simulink model "task4_final"  (R2019b)
settings: Solver=ode45  StartTime=0.0  StopTime=10.0  RelTol=1e-3  EnableMultiTasking=on
settings Model: Creator=Knut  LastModifiedBy=FFARHANW
settings DataIOCC: LimitDataPoints=on  SaveFormat=Array  SignalLoggingSaveFormat=ModelDataLogs  ReturnWorkspaceOutputs=off
settings OptimizationCC: BlockReduction=off  BooleanDataType=off
settings DebuggingCC: SaveWithParameterizedLinksMsg=none  UnderspecifiedInitializationDetection=Classic  MergeDetectMultiDrivingBlocksExec=none  SignalResolutionControl=TryResolveAllWithWarning  MultiTaskDSMMsg=warning  MultiTaskCondExecSysMsg=none  ArithmeticOperatorsInVariantConditions=warning
settings HardwareCC: TargetUnknown=on
settings ModelReferenceCC: PropagateSignalLabelsOutOfModel=off
settings SFSimCC: SimUseLocalCustomCode=off  CustomCodeUndefinedFunction=UseInterfaceOnly
settings RTWCC: RTWUseLocalCustomCode=off
settings CodeAppCC: StateflowObjectComments=on
settings GRTTargetCC: TargetLangStandard=C89/C90 (ANSI)  CombineOutputUpdateFcns=off  GRTInterface=on
settings ConfigComp: CovHtmlReporting=on  CovSaveCumulativeToWorkspaceVar=on  CovSaveSingleToWorkspaceVar=on  CovExternalEMLEnable=off

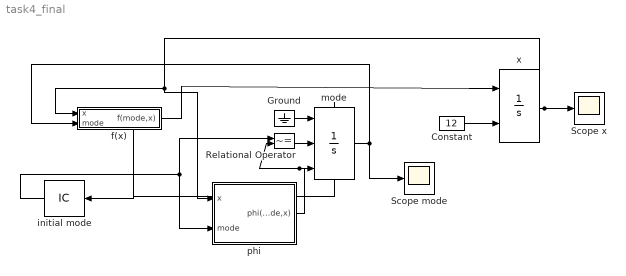
== system task4_final ==
  Constant : Constant  Value=12
  Ground : Ground
  Relational Operator : RelationalOperator  Operator=~=  RndMeth=Nearest  InputSameDT=on
  Scope mode : Scope
  Scope x : Scope
  f(x) : Subsystem  Description=f(x)
  initial mode : InitialCondition
  mode : Integrator  ExternalReset=rising  InitialConditionSource=external  ShowStatePort=on  ZeroCross=off
  phi : Subsystem  Description=f(x)
  x : Integrator  InitialConditionSource=external  LowerSaturationLimit=0
  wires:
  f(x)/1(f(mode,x)) -> x/1
  Ground/1 -> mode/1
  mode/State -> initial mode/1
  initial mode/1 -> phi/2(mode), Relational Operator/1
  mode/1 -> Scope mode/1, f(x)/2(mode)
  phi/1(phi(mode,x)) -> Relational Operator/2, mode/3
  x/1 -> phi/1(x), f(x)/1(x), Scope x/1
  Relational Operator/1 -> mode/2
  Constant/1 -> x/2

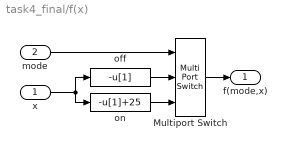
== system task4_final/f(x) ==
  x : Inport
  mode : Inport  Port=2
  Multiport Switch : MultiPortSwitch  Inputs=2  SaturateOnIntegerOverflow=on  InputSameDT=on
  off : Fcn  Expr=-u[1]
  on : Fcn  Expr=-u[1]+25
  f(mode,x) : Outport
  wires:
  Multiport Switch/1 -> f(mode,x)/1
  off/1 -> Multiport Switch/2
  on/1 -> Multiport Switch/3
  x/1 -> off/1, on/1
  mode/1 -> Multiport Switch/1

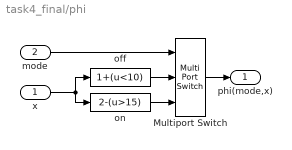
== system task4_final/phi ==
  x : Inport
  mode : Inport  Port=2
  Multiport Switch : MultiPortSwitch  Inputs=2  SaturateOnIntegerOverflow=on  InputSameDT=on
  off : Fcn  Expr=1+(u<10)
  on : Fcn  Expr=2-(u>15)
  phi(mode,x) : Outport
  wires:
  x/1 -> on/1, off/1
  on/1 -> Multiport Switch/3
  off/1 -> Multiport Switch/2
  Multiport Switch/1 -> phi(mode,x)/1
  mode/1 -> Multiport Switch/1
